simulink model "pendcart"  (Simulink 8.9)
settings: Solver=ode45  StartTime=0.0  StopTime=tsim  RelTol=1e-3  EnableMultiTasking=on
values from neighbouring files (symbols this model uses):
  eta = 0.5882    [testmotor.m]
  I = u(8)    [massMat.m]    (also in pendcartsim.m = 0.0625)
  J = u(1)    [massMat.m]    (also in pendcartsim.m = 0.0018375)
  K = 0.1    [pendcartsim.m]    (also in testmotor.m)
  Kgain = place(Ad,Bd,[-15 -16 -17])    [pendcartsim.m]
  l = u(3)    [ElementMatrix.m]    (also in massMat.m = u(7); pendcartsim.m = 0.5)
  L = 0.001    [pendcartsim.m]
  M = u(2)    [ElementMatrix.m]    (also in massMat.m; pendcartsim.m = 3)
  m = u(8)    [ElementMatrix.m]    (also in massMat.m = u(3); pendcartsim.m = 0.5)
  N = 50    [pendcartsim.m]    (also in testmotor.m)
  Ngain = 1/(Cd*inv(eye(3)-Ad+Bd*Kgain)*Bd)    [pendcartsim.m]
  r = u(4)    [ElementMatrix.m]    (also in massMat.m; pendcartsim.m = 0.035; testmotor.m = 0.035)
  R = 0.6575    [pendcartsim.m]    (also in testmotor.m)
  taum = 0.0056    [pendcartsim.m]    (also in testmotor.m)
  theta0 = 10*pi/180    (= 0.174532925199)    [pendcartsim.m]
settings Model: Creator=Chris  LastModifiedBy=Dell
settings OptimizationCC: ExpressionDepthLimit=2147483647  InitFltsAndDblsToZero=on
settings DebuggingCC: AlgebraicLoopMsg=none  SaveWithParameterizedLinksMsg=none  AllowSymbolicDim=off
settings GRTTargetCC: TargetFcnLib=ansi_tfl_tmw.mat

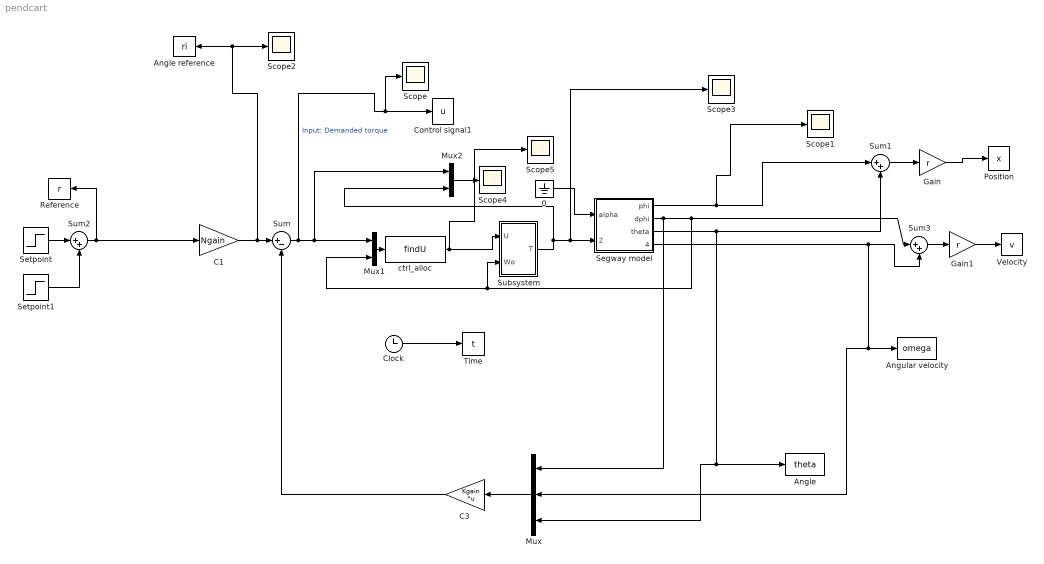
== system pendcart ==
  0 : Ground
  Angle : ToWorkspace  VariableName=theta  SampleTime=-1
  Angle reference : ToWorkspace  VariableName=ri  SampleTime=-1
  Angular velocity : ToWorkspace  VariableName=omega  SampleTime=-1
  C1 : Gain  Gain=Ngain
  C3 : Gain  Gain=Kgain  Multiplication=Matrix(K*u)
  Clock : Clock
  Control signal1 : ToWorkspace  VariableName=u  SampleTime=-1
  Gain : Gain  Gain=r
  Gain1 : Gain  Gain=r
  Mux : Mux  Inputs=3
  Mux1 : Mux  Inputs=2
  Mux2 : Mux  Inputs=2
  Position : ToWorkspace  VariableName=x  SampleTime=-1
  Reference : ToWorkspace  VariableName=r  SampleTime=-1
  Scope{,1..5} (6 alike) : Scope
  Segway model : Subsystem
  Setpoint : Step  Time=10  After=0.5  SampleTime=0
  Setpoint1 : Step  Time=20  After=-0.5  SampleTime=0
  Subsystem : Subsystem
  Sum : Sum  Inputs=|+-
  Sum1 : Sum  Inputs=|++
  Sum2 : Sum  Inputs=|++
  Sum3 : Sum  Inputs=|++
  Time : ToWorkspace  VariableName=t  SampleTime=-1
  Velocity : ToWorkspace  VariableName=v  SampleTime=-1
  ctrl_alloc : MATLABFcn  MATLABFcn=findU
  wires:
  Clock/1 -> Time/1
  Segway model/1(phi) -> Sum1/1, Scope1/1
  Sum/1 -> Scope/1, Control signal1/1, Mux2/1, Mux1/1  "Input: Demanded torque"
  Segway model/2(dphi) -> Mux1/2, Subsystem/2(Wo), Sum3/1, Mux/1
  Segway model/3(theta) -> Mux/3, Angle/1, Sum1/2
  Setpoint/1 -> Sum2/1
  Setpoint1/1 -> Sum2/2
  0/1 -> Segway model/1(alpha)
  C3/1 -> Sum/2
  Mux/1 -> C3/1
  Segway model/4(omega) -> Mux/2, Angular velocity/1, Sum3/2
  Gain/1 -> Position/1
  Sum1/1 -> Gain/1
  Sum3/1 -> Gain1/1
  C1/1 -> Angle reference/1, Scope2/1, Sum/1
  Sum2/1 -> C1/1, Reference/1
  Mux1/1 -> ctrl_alloc/1
  Subsystem/1(T) -> Mux2/2, Segway model/2(Torque), Scope3/1
  Gain1/1 -> Velocity/1
  Mux2/1 -> Scope4/1
  ctrl_alloc/1 -> Subsystem/1(U), Scope5/1

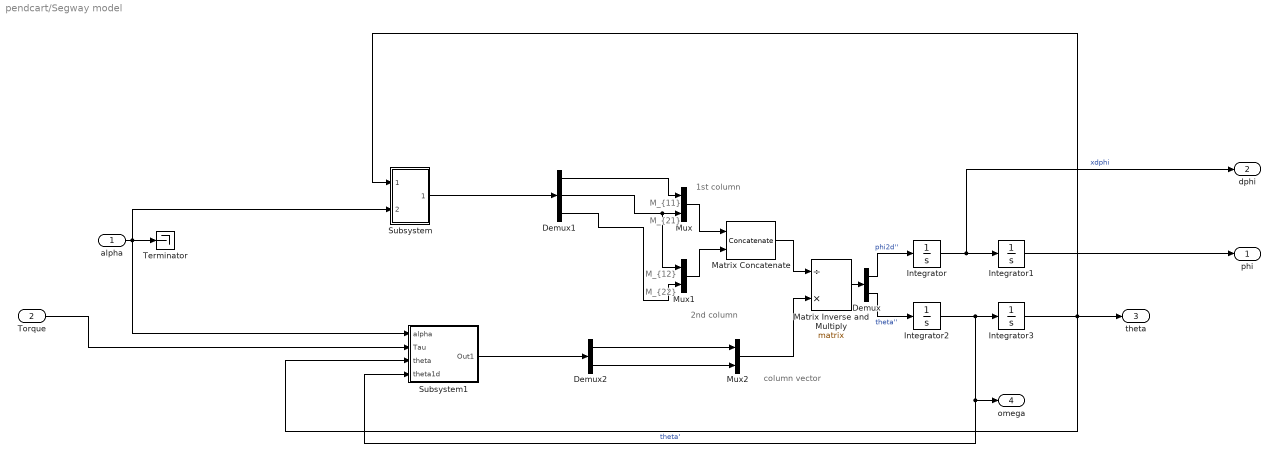
== system pendcart/Segway model ==
  note: M_{11}
  note: M_{21}
  note: M_{12}
  note: M_{22}
  note: 1st column
  note: 2nd column
  note: column vector
  alpha : Inport
  Torque : Inport  Port=2
  Demux : Demux  Outputs=2
  Demux1 : Demux  Outputs=3
  Demux2 : Demux  Outputs=2
  Integrator : Integrator
  Integrator1 : Integrator
  Integrator2 : Integrator
  Integrator3 : Integrator  InitialCondition=theta0
  Matrix Concatenate : Concatenate  Mode=Multidimensional array  ConcatenateDimension=2
  Matrix Inverse and Multiply : Product  Inputs=/*  Multiplication=Matrix(*)
  Mux : Mux  Inputs=2
  Mux1 : Mux  Inputs=2
  Mux2 : Mux  Inputs=2
  Subsystem : Subsystem
  Subsystem1 : Subsystem
  Terminator : Terminator
  phi : Outport
  dphi : Outport  Port=2
  theta : Outport  Port=3
  omega : Outport  Port=4
  wires:
  Demux/1 -> Integrator/1  "phi2d''"
  Integrator/1 -> dphi/1, Integrator1/1  "xdphi"
  Demux/2 -> Integrator2/1  "theta''"
  Integrator2/1 -> Integrator3/1, Subsystem1/4(theta1d), omega/1  "theta'"
  Matrix Inverse and Multiply/1 -> Demux/1
  Mux1/1 -> Matrix Concatenate/2
  Mux/1 -> Matrix Concatenate/1
  Matrix Concatenate/1 -> Matrix Inverse and Multiply/1
  Mux2/1 -> Matrix Inverse and Multiply/2
  alpha/1 -> Subsystem1/1(alpha), Subsystem/2(alpha), Terminator/1
  Integrator3/1 -> Subsystem1/3(theta), Subsystem/1(theta), theta/1
  Demux1/3 -> Mux1/2
  Demux1/2 -> Mux/2, Mux1/1
  Demux1/1 -> Mux/1
  Subsystem/1(Out1) -> Demux1/1
  Demux2/1 -> Mux2/1
  Demux2/2 -> Mux2/2
  Torque/1 -> Subsystem1/2(Tau)
  Subsystem1/1(Out1) -> Demux2/1
  Integrator1/1 -> phi/1

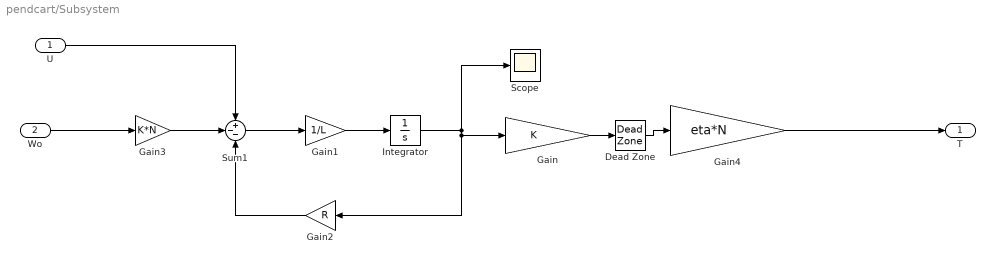
== system pendcart/Subsystem ==
  U : Inport
  Wo : Inport  Port=2
  Dead Zone : DeadZone  LowerValue=-taum  UpperValue=taum  SaturateOnIntegerOverflow=on
  Gain : Gain  Gain=K
  Gain1 : Gain  Gain=1/L
  Gain2 : Gain  Gain=R
  Gain3 : Gain  Gain=K*N
  Gain4 : Gain  Gain=eta*N
  Integrator : Integrator
  Scope : Scope
  Sum1 : Sum  Inputs=+--
  T : Outport
  wires:
  Integrator/1 -> Gain2/1, Gain/1, Scope/1
  Gain2/1 -> Sum1/3
  Gain1/1 -> Integrator/1
  U/1 -> Sum1/1
  Wo/1 -> Gain3/1
  Gain3/1 -> Sum1/2
  Gain/1 -> Dead Zone/1
  Sum1/1 -> Gain1/1
  Dead Zone/1 -> Gain4/1
  Gain4/1 -> T/1

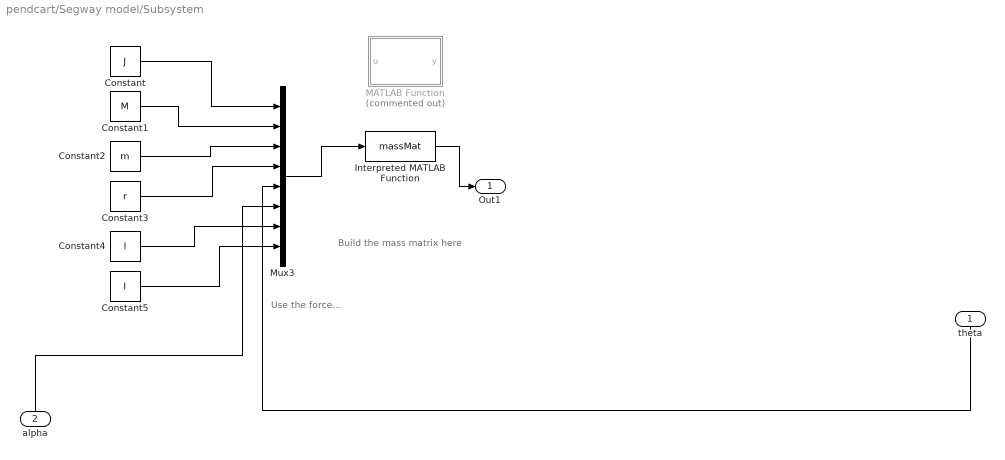
== system pendcart/Segway model/Subsystem ==
  note: Build the mass matrix here
  note: Use the force...
  theta : Inport
  alpha : Inport  Port=2
  Constant : Constant  Value=J
  Constant1 : Constant  Value=M
  Constant2 : Constant  Value=m
  Constant3 : Constant  Value=r
  Constant4 : Constant  Value=l
  Constant5 : Constant  Value=I
  Interpreted MATLAB Function : MATLABFcn  MATLABFcn=massMat
  MATLAB Function : MATLAB Function  Commented=on  TreatAsAtomicUnit=on
  Mux3 : Mux  Inputs=8
  Out1 : Outport
  wires:
  alpha/1 -> Mux3/6
  theta/1 -> Mux3/5
  Constant5/1 -> Mux3/8
  Interpreted MATLAB Function/1 -> Out1/1
  Constant4/1 -> Mux3/7
  Mux3/1 -> Interpreted MATLAB Function/1
  Constant3/1 -> Mux3/4
  Constant/1 -> Mux3/1
  Constant1/1 -> Mux3/2
  Constant2/1 -> Mux3/3

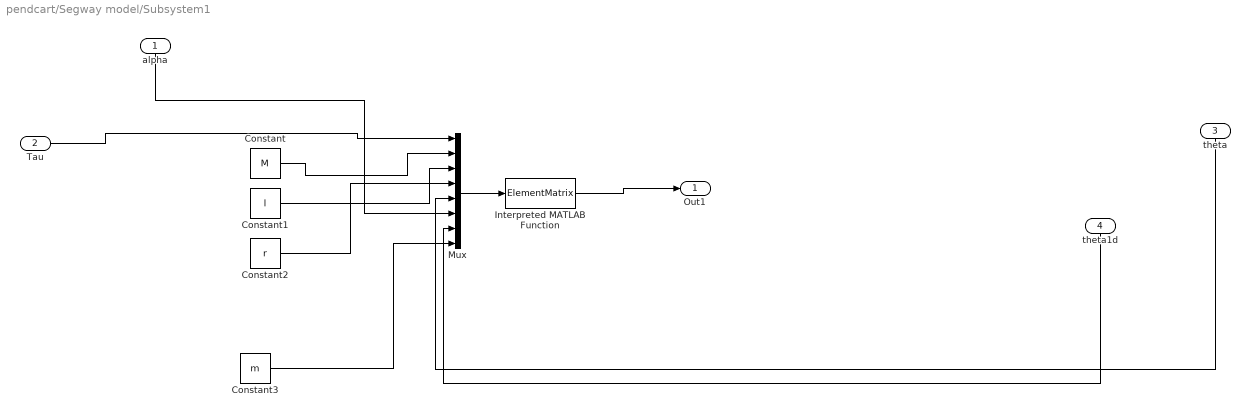
== system pendcart/Segway model/Subsystem1 ==
  alpha : Inport
  Tau : Inport  Port=2
  theta : Inport  Port=3
  theta1d : Inport  Port=4
  Constant : Constant  Value=M
  Constant1 : Constant  Value=l
  Constant2 : Constant  Value=r
  Constant3 : Constant  Value=m
  Interpreted MATLAB Function : MATLABFcn  MATLABFcn=ElementMatrix
  Mux : Mux  Inputs=8
  Out1 : Outport
  wires:
  Constant/1 -> Mux/2
  Tau/1 -> Mux/1
  Constant3/1 -> Mux/8
  Interpreted MATLAB Function/1 -> Out1/1
  theta/1 -> Mux/5
  theta1d/1 -> Mux/7
  alpha/1 -> Mux/6
  Constant2/1 -> Mux/4
  Constant1/1 -> Mux/3
  Mux/1 -> Interpreted MATLAB Function/1

== matlab function Segway model/Subsystem/MATLAB Function ==
  data: u input double; y output double
function y = fcn(u)
%#codegen
J = u(1);
M = u(2);
m = u(3);
r = u(4);
theta = u(5);
alpha = u(6);
l = u(7);
I = u(8);



M11 = J + (M+m)*r^2;
M12 = J + (M+m)*r^2 + M*l*r*cos(theta+alpha);
M22 = J + (M+m)*r^2 + 2*M*l*r*cos(theta+alpha) + I + M*l^2;
y = [M11;M12;M22];
